simulink model "firfilter"  (R2020a)
settings: Solver=VariableStepAuto  StartTime=0.0  StopTime=10.0  RelTol=1e-3
libraries: simulink x1
settings Model: Creator=Admin  LastModifiedBy=Admin

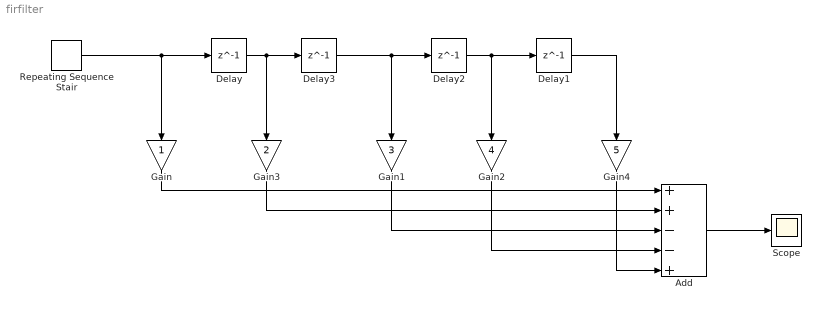
== system firfilter ==
  Add : Sum  Inputs=++--+
  Delay{,1..3} (4 alike) : Delay  DelayLength=1
  Gain : Gain
  Gain1 : Gain  Gain=3
  Gain2 : Gain  Gain=4
  Gain3 : Gain  Gain=2
  Gain4 : Gain  Gain=5
  Repeating Sequence Stair : simulink/Sources/Repeating Sequence Stair  OutValues=[3 1 4 2 1].'  tsamp=-1  OutMin=[]  OutMax=[]  OutDataTypeStr=double  OutputDataTypeScalingMode=double  OutDataType=fixdt(0,8)  ConRadixGroup=Best Precision: Vector-wise  OutScaling=2^-12
  Scope : Scope
  wires:
  Delay/1 -> Gain3/1, Delay3/1
  Delay3/1 -> Gain1/1, Delay2/1
  Delay2/1 -> Gain2/1, Delay1/1
  Delay1/1 -> Gain4/1
  Repeating Sequence Stair/1 -> Delay/1, Gain/1
  Gain4/1 -> Add/5
  Gain2/1 -> Add/4
  Gain1/1 -> Add/3
  Gain3/1 -> Add/2
  Gain/1 -> Add/1
  Add/1 -> Scope/1
